simulink model "sl_tripleangle"  (R2018a)
settings: Solver=VariableStepAuto  StartTime=0.0  StopTime=1  RelTol=1e-3
libraries: roblocks x4
settings Model: Creator=corkep  LastModifiedBy=corkep
settings DataIOCC: SaveFormat=Structure  SignalLogging=off  DSMLogging=off  SaveTime=off

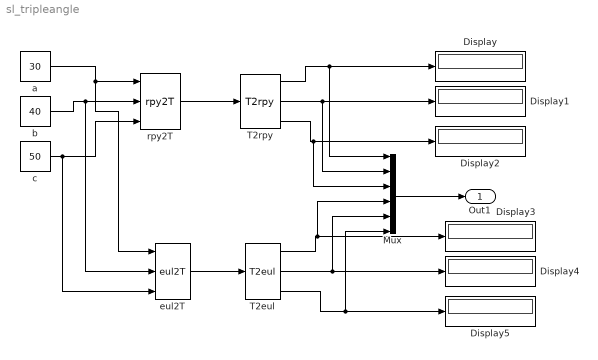
== system sl_tripleangle ==
  Display{,1..5} (6 alike) : Display
  Mux : Mux  Inputs=6
  T2eul : roblocks/Toolbox/T2eul  degrees=on
  T2rpy : roblocks/Toolbox/T2rpy  sequence=YXZ  degrees=on
  a : Constant  Value=30
  b : Constant  Value=40
  c : Constant  Value=50
  eul2T : roblocks/Toolbox/eul2T  degrees=on
  rpy2T : roblocks/Toolbox/rpy2T  sequence=YXZ  degrees=on
  Out1 : Outport
  wires:
  rpy2T/1 -> T2rpy/1
  a/1 -> eul2T/1, rpy2T/1
  c/1 -> eul2T/3, rpy2T/3
  b/1 -> eul2T/2, rpy2T/2
  T2rpy/1 -> Mux/1, Display/1
  T2rpy/2 -> Mux/2, Display1/1
  T2rpy/3 -> Mux/3, Display2/1
  T2eul/3 -> Mux/6, Display5/1
  T2eul/1 -> Mux/4, Display3/1
  T2eul/2 -> Mux/5, Display4/1
  eul2T/1 -> T2eul/1
  Mux/1 -> Out1/1
